simulink model "pendulum_Kapitsa"  (R2020a)
settings: Solver=VariableStepAuto  StartTime=0.0  StopTime=15.0  MaxStep=0.01  RelTol=1e-3
values from neighbouring files (symbols this model uses):
  A = 0.1    [script_pendulum_Kapitsa.m]
  F = 5    [script_pendulum_Kapitsa.m]    (also in script_pendulum_cart.m = 0.2)
libraries: simulink_extras x1, simulink x1
settings Model: Creator=kiril_000  LastModifiedBy=kiril_000

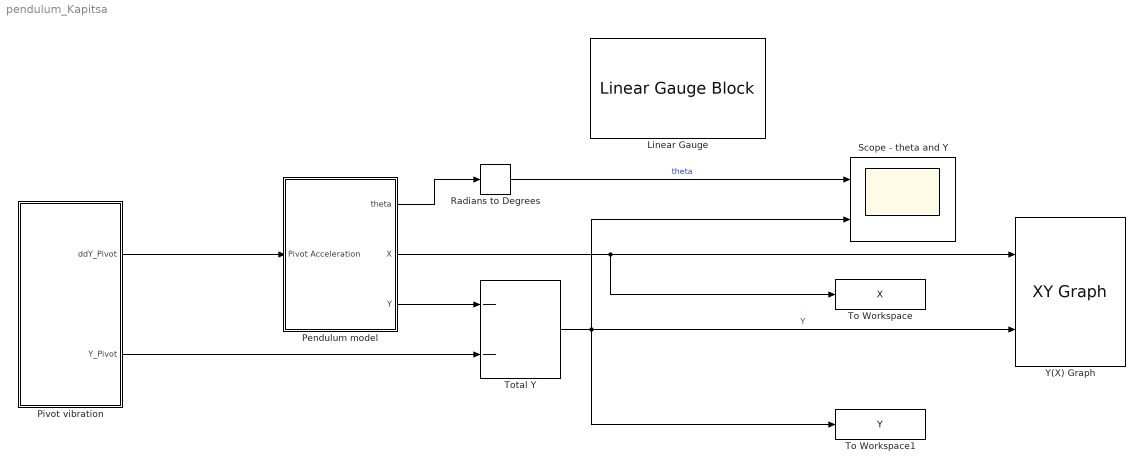
== system pendulum_Kapitsa ==
  Linear Gauge : LinearGaugeBlock  ScaleMin=-90  ScaleMax=90
  Pendulum model : Subsystem  mask{m=1, l=1, g=9.8, b=0.5}
      mask prompts: m "Масса"; l "Длина"; g "Ускорение свободного падения"; b "Коэффициент вязкости"
      mask init:
      | I = m * l^2
  Pivot vibration : Subsystem  mask{A=A, F=F}
  Radians to Degrees : simulink_extras/Transformations/Radians to Degrees
  Scope - theta and Y : Scope  NumInputPorts=2
  To Workspace : ToWorkspace  VariableName=X  SampleTime=-1
      settings: Save2DSignal=2-D array (concatenate along first dimension)
  To Workspace1 : ToWorkspace  VariableName=Y  SampleTime=-1
      settings: Save2DSignal=2-D array (concatenate along first dimension)
  Total Y : Sum  Inputs=--
  Y(X) Graph : simulink/Sinks/XY Graph  xmin=-1  xmax=1  ymin=-3  ymax=3  st=-1
  wires:
  Pendulum model/1(theta) -> Radians to Degrees/1
  Radians to Degrees/1 -> Scope - theta and Y/1  "theta"
  Pivot vibration/1(ddY_Pivot) -> Pendulum model/1(Pivot Acceleration)
  Pendulum model/2(X) -> To Workspace/1, Y(X) Graph/1
  Pivot vibration/2(Y_Pivot) -> Total Y/2
  Pendulum model/3(Y) -> Total Y/1
  Total Y/1 -> Scope - theta and Y/2, Y(X) Graph/2, To Workspace1/1  "Y"

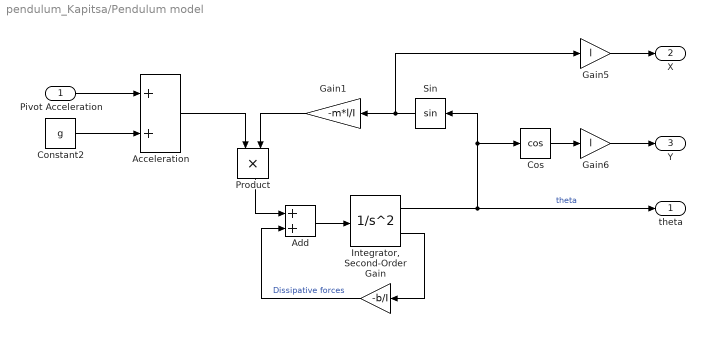
== system pendulum_Kapitsa/Pendulum model ==
  Pivot Acceleration : Inport
  Acceleration : Sum
  Add : Sum
  Constant2 : Constant  Value=g
  Cos : Trigonometry  Operator=cos
  Gain : Gain  Gain=-b/I
  Gain1 : Gain  Gain=-m*l/I
  Gain5 : Gain  Gain=l
  Gain6 : Gain  Gain=l
  "Integrator, Second-Order" : SecondOrderIntegrator  ICX=deg2rad(135)
  Product : Product
  Sin : Trigonometry
  theta : Outport
  X : Outport  Port=2
  Y : Outport  Port=3
  wires:
  Sin/1 -> Gain1/1, Gain5/1
  "Integrator, Second-Order"/2 -> Gain/1
  "Integrator, Second-Order"/1 -> Cos/1, Sin/1, theta/1  "theta"
  Gain1/1 -> Product/2
  Add/1 -> "Integrator, Second-Order"/1
  Gain/1 -> Add/2  "Dissipative forces"
  Cos/1 -> Gain6/1
  Pivot Acceleration/1 -> Acceleration/1
  Constant2/1 -> Acceleration/2
  Acceleration/1 -> Product/1
  Product/1 -> Add/1
  Gain5/1 -> X/1
  Gain6/1 -> Y/1

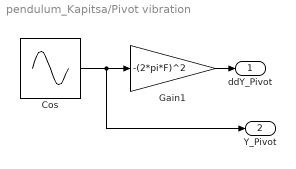
== system pendulum_Kapitsa/Pivot vibration ==
  Cos : Sin  Amplitude=A  Frequency=2*pi*F  Phase=pi/2  SampleTime=0
  Gain1 : Gain  Gain=-(2*pi*F)^2
  ddY_Pivot : Outport
  Y_Pivot : Outport  Port=2
  wires:
  Cos/1 -> Y_Pivot/1, Gain1/1
  Gain1/1 -> ddY_Pivot/1
